simulink model "accelerometer"  (R2019a)
settings: Solver=FixedStepAuto  StartTime=0.0  StopTime=inf  RelTol=1e-3  EnableMultiTasking=on
libraries: raspberrypilib x3
settings Model: SimulationMode=external  Creator=florian  LastModifiedBy=florian
settings SolverCC: PositivePriorityOrder=on
settings OptimizationCC: EnhancedBackFolding=on  PassReuseOutputArgsAs=Individual arguments  MaxStackSize=64  OptimizeBlockOrder=speed  DifferentSizesBufferReuse=on  OptimizationCustomize=off
settings DebuggingCC: ParameterTunabilityLossMsg=error
settings HardwareCC: ProdBitPerPointer=32  ProdBitPerSizeT=32  ProdBitPerPtrDiffT=32  ProdLargestAtomicInteger=Long  ProdLargestAtomicFloat=Double  ProdWordSize=32  ProdLongLongMode=on  ProdHWDeviceType=ARM Compatible->ARM Cortex
settings SFSimCC: MATLABDynamicMemAlloc=off
settings RTWCC: SystemTargetFile=ert.tlc  HardwareBoard=Raspberry Pi  TLCOptions="-aInlineSetEventsForThisBaseRateFcn=TLC_FALSE -aSuppressMultiTaskScheduler=TLC_FALSE  -aRateBasedStepFcn=0"  TemplateMakefile=ert_default_tmf  GenerateReport=on  Toolchain=GNU GCC Raspberry Pi  BuildConfiguration=Faster Runs  IncludeHyperlinkInReport=on  LaunchReport=on  GenerateTraceInfo=on  GenerateTraceReport=on  GenerateTraceReportSl=on  GenerateTraceReportSf=on  GenerateTraceReportEml=on
settings CodeAppCC: ForceParamTrailComments=on  IgnoreCustomStorageClasses=off  OperatorAnnotations=on  SimulinkDataObjDesc=on  SFDataObjDesc=on  InsertBlockDesc=on
settings ERTTargetCC: SupportVariableSizeSignals=on

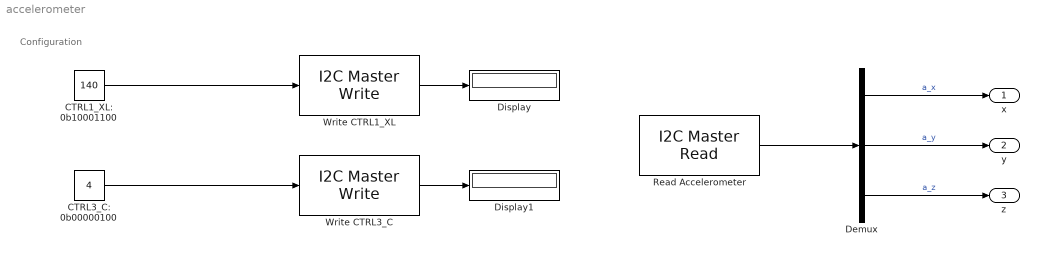
== system accelerometer ==
  note: Configuration
  CTRL1_XL: 0b10001100 : Constant  Priority=0  Value=140  OutDataTypeStr=uint8
  CTRL3_C: 0b00000100 : Constant  Value=4  OutDataTypeStr=uint8
  Demux : Demux  Outputs=3
  Display : Display
  Display1 : Display
  Read Accelerometer : raspberrypilib/I2C Master Read  Priority=1  BoardProperty=Pi 3 Model B+  Mode=Master  SlaveAddress=107  SlaveByteOrder=LittleEndian  Direction=Receiver  RegisterAddressMode=on  RegisterAddress=40  SlaveDataType=int16  DataLength=3  NoAck=off  RepeatedStart=off  OutputStatus=off  SampleTime=0.01
      settings: SourceProductName=Simulink Support Package for Raspberry Pi Hardware  SourceProductBaseCode=RASPPI
  Write CTRL1_XL : raspberrypilib/I2C Master Write  Priority=0  BoardProperty=Pi 3 Model B+  Mode=Master  SlaveAddress=107  SlaveByteOrder=LittleEndian  Direction=Transmitter  RegisterAddressMode=on  RegisterAddress=16  SlaveDataType=uint8  DataLength=1  NoAck=off  RepeatedStart=off  OutputStatus=on
      settings: SourceProductName=Simulink Support Package for Raspberry Pi Hardware  SourceProductBaseCode=RASPPI
  Write CTRL3_C : raspberrypilib/I2C Master Write  Priority=0  BoardProperty=Pi 3 Model B+  Mode=Master  SlaveAddress=107  SlaveByteOrder=LittleEndian  Direction=Transmitter  RegisterAddressMode=on  RegisterAddress=18  SlaveDataType=uint8  DataLength=1  NoAck=off  RepeatedStart=off  OutputStatus=on
      settings: SourceProductName=Simulink Support Package for Raspberry Pi Hardware  SourceProductBaseCode=RASPPI
  x : Outport
  y : Outport  Port=2
  z : Outport  Port=3
  wires:
  Demux/1 -> x/1  "a_x"
  CTRL3_C: 0b00000100/1 -> Write CTRL3_C/1
  CTRL1_XL: 0b10001100/1 -> Write CTRL1_XL/1
  Demux/3 -> z/1  "a_z"
  Demux/2 -> y/1  "a_y"
  Read Accelerometer/1 -> Demux/1
  Write CTRL1_XL/1 -> Display/1
  Write CTRL3_C/1 -> Display1/1
